simulink model "Imitator_controller"  (R2019b)
settings: Solver=ode4  StartTime=0.0  StopTime=0.6  FixedStep=1e-6  MaxStep=1  RelTol=1e-3  EnableMultiTasking=on
InitFcn:
  | %initialization file
  | clear
  | Rl=0.1;
  | Rload=60;
  | L=2.4e-3;
  | C=14e-6;
  | wref=2*pi*50;
  | Vdc=700;
  | Ts=20e-6;
  | s=tf('s');
  | Vac=325;
  | Td=4e-6;
  | 
  | %net = importKerasNetwork('model_9796.h5','Classes',{'State 1', 'State 2', 'State 3', 'State 4', 'State 5', 'State 6', 'State 7'});
  | %weights1 = double(net.Layers(2,1).Weights);
  | %biases1 = double(net.Layers(2,1).Bias);
  | %weights2 =double(net.Layers(4,1).Weights);
  | %biases2 = double(net.Layers(4,1).Bias);
  | 
  | weights1 = load('weights1.mat');
  | weights1 = weights1.weights1;
  | weights2 = load('weights2.mat');
  | weights2 = weights2.weights2;
  | biases1 = load('biases1.mat');
  | biases1 = biases1.biases1;
  | biases2 = load('biases2.mat');
  | biases2 = biases2.biases2;
undefined symbols (not defined in the file): Lc, Lload, plecs
libraries: neural x95, powerlib x18, powerlib_meascontrol x4
(part 4 of 4)

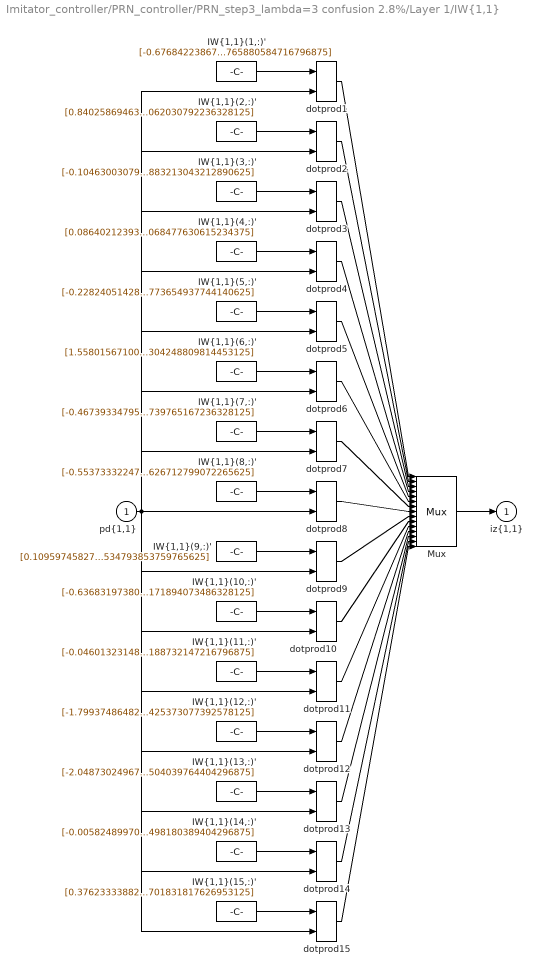
== system Imitator_controller/PRN_controller/PRN_step3_lambda=3 confusion 2.8%/Layer 1/IW{1,1} ==
  "pd{1,1}" : Inport  PortDimensions=8
      mask Display: e = 0.06;c1 = [120 230 180]/255;c2 = ([120 230 180]+0)/(256+128);c3 = ([120 230 180]+128)/(256+128);patch([0 1 1 0],[0 0 1 1],c1);patch([0 1 1 1-e 1-e 0+e],[0 0 1 1-e 0+e 0+e],c2);patch([0 0 1 1-e 0+e 0+e],[0 1 1 1-e 1-e 0+e],c3);plot([0 1 1 0 0],[0 0 1 1 0]);
  "IW{1,1}(1,:)'" : Constant  Value=[-0.676842238677143104297329045948572456836700439453125;-1.9888159175228456998496540109044872224330902099609375;0.73765036780827186735365330605418421328067779541015625;1.71320701226988081344870806788094341754913330078125;0.038398725205589963327401648029990610666573047637939453125;0.04866552570600853055982071282414835877716541290283203125;0.26518608289125467081248643808066844940185546875;-0.19441986416535694814911039429716765880584716796875]
      mask Display: e = 0.06;c1 = [120 150 230]/255;c2 = ([120 150 230]+0)/383;c3 = ([120 150 230]+128)/383;patch([0 1 1 0],[0 0 1 1],c1);patch([0 1 1 1-e 1-e 0+e],[0 0 1 1-e 0+e 0+e],c2);patch([0 0 1 1-e 0+e 0+e],[0 1 1 1-e 1-e 0+e],c3);plot([0 1 1 0 0],[0 0 1 1 0]);disp('Weights');
  "IW{1,1}(10,:)'" : Constant  Value=[-0.63683197380668221665445116741466335952281951904296875;-0.11544459149383486107343088633570005185902118682861328125;-0.36758148612573238178669043918489478528499603271484375;-0.0678774326477270262270025114048621617257595062255859375;-0.046861816789189041088103948595744441263377666473388671875;-0.0058226912142529119176259655432659201323986053466796875;-0.02697450161674534718780904540835763327777385711669921875;1.247120666092144336545288751949556171894073486328125]
      mask Display: e = 0.06;c1 = [120 150 230]/255;c2 = ([120 150 230]+0)/383;c3 = ([120 150 230]+128)/383;patch([0 1 1 0],[0 0 1 1],c1);patch([0 1 1 1-e 1-e 0+e],[0 0 1 1-e 0+e 0+e],c2);patch([0 0 1 1-e 0+e 0+e],[0 1 1 1-e 1-e 0+e],c3);plot([0 1 1 0 0],[0 0 1 1 0]);disp('Weights');
  "IW{1,1}(11,:)'" : Constant  Value=[-0.0460132314806563080811230292965774424374103546142578125;0.01473816958439077250131443719283197424374520778656005859375;0.055555128220495651747423693223026930354535579681396484375;0.049792053782768734560004730838045361451804637908935546875;0.004235491339451513854996722585610768874175846576690673828125;0.003769159624020011235823179873705157660879194736480712890625;-2.82485738553735021838519969605840742588043212890625;-0.01265950989853382828431715978467764216475188732147216796875]
      mask Display: e = 0.06;c1 = [120 150 230]/255;c2 = ([120 150 230]+0)/383;c3 = ([120 150 230]+128)/383;patch([0 1 1 0],[0 0 1 1],c1);patch([0 1 1 1-e 1-e 0+e],[0 0 1 1-e 0+e 0+e],c2);patch([0 0 1 1-e 0+e 0+e],[0 1 1 1-e 1-e 0+e],c3);plot([0 1 1 0 0],[0 0 1 1 0]);disp('Weights');
  "IW{1,1}(12,:)'" : Constant  Value=[-1.7993748648200000861407943375525064766407012939453125;0.1476111476191077909181359473222983069717884063720703125;2.35416836327518108618050973745994269847869873046875;-0.00120452360425208466164492815408948445110581815242767333984375;0.11793391068665191878661602231659344397485256195068359375;0.00113378894210611311406389223321866666083224117755889892578125;1.7721939806664346317433000876917503774166107177734375;-0.268337504582858266122258328323368914425373077392578125]
      mask Display: e = 0.06;c1 = [120 150 230]/255;c2 = ([120 150 230]+0)/383;c3 = ([120 150 230]+128)/383;patch([0 1 1 0],[0 0 1 1],c1);patch([0 1 1 1-e 1-e 0+e],[0 0 1 1-e 0+e 0+e],c2);patch([0 0 1 1-e 0+e 0+e],[0 1 1 1-e 1-e 0+e],c3);plot([0 1 1 0 0],[0 0 1 1 0]);disp('Weights');
  "IW{1,1}(13,:)'" : Constant  Value=[-2.04873024967913952565368163050152361392974853515625;0.1439969197044075333025148211163468658924102783203125;2.577017004086017859521007267176173627376556396484375;0.0318978273732246353500130453539895825088024139404296875;0.11836244796372562271269401890094741247594356536865234375;0.002369781613885219191673048300117443432100117206573486328125;1.8033596226591666056293661313247866928577423095703125;-0.55506848791334906234595791829633526504039764404296875]
      mask Display: e = 0.06;c1 = [120 150 230]/255;c2 = ([120 150 230]+0)/383;c3 = ([120 150 230]+128)/383;patch([0 1 1 0],[0 0 1 1],c1);patch([0 1 1 1-e 1-e 0+e],[0 0 1 1-e 0+e 0+e],c2);patch([0 0 1 1-e 0+e 0+e],[0 1 1 1-e 1-e 0+e],c3);plot([0 1 1 0 0],[0 0 1 1 0]);disp('Weights');
  "IW{1,1}(14,:)'" : Constant  Value=[-0.005824899707417730866654270727167386212386190891265869140625;-0.00300316480099391096281191693151413346640765666961669921875;0.03114520666426491557476907701129675842821598052978515625;0.006670702704397522657397967549286477151326835155487060546875;-0.000317029194644610572660636815811585620394907891750335693359375;-0.0004181329362500792417960127078657706078956834971904754638671875;-4.56994739529403926070472152787260711193084716796875;0.0021206975737620421644524792981201244401745498180389404296875]
      mask Display: e = 0.06;c1 = [120 150 230]/255;c2 = ([120 150 230]+0)/383;c3 = ([120 150 230]+128)/383;patch([0 1 1 0],[0 0 1 1],c1);patch([0 1 1 1-e 1-e 0+e],[0 0 1 1-e 0+e 0+e],c2);patch([0 0 1 1-e 0+e 0+e],[0 1 1 1-e 1-e 0+e],c3);plot([0 1 1 0 0],[0 0 1 1 0]);disp('Weights');
  "IW{1,1}(15,:)'" : Constant  Value=[0.3762333388259329058911362153594382107257843017578125;1.9877672677136974943579161845264025032520294189453125;-0.4572160922242147762517561204731464385986328125;-1.909758831917812482714680299977771937847137451171875;-0.01745565839131461849387250140352989546954631805419921875;-0.07136074826339115773077281801306526176631450653076171875;-1.0942687606048513426770796286291442811489105224609375;0.0170705351700497949540835662673998740501701831817626953125]
      mask Display: e = 0.06;c1 = [120 150 230]/255;c2 = ([120 150 230]+0)/383;c3 = ([120 150 230]+128)/383;patch([0 1 1 0],[0 0 1 1],c1);patch([0 1 1 1-e 1-e 0+e],[0 0 1 1-e 0+e 0+e],c2);patch([0 0 1 1-e 0+e 0+e],[0 1 1 1-e 1-e 0+e],c3);plot([0 1 1 0 0],[0 0 1 1 0]);disp('Weights');
  "IW{1,1}(2,:)'" : Constant  Value=[0.8402586946382888388740184382186271250247955322265625;2.9740480510521773993559691007249057292938232421875;-0.87581495641554429898434364076820202171802520751953125;-2.58606131308167608295889294822700321674346923828125;-0.044568205229961764535229207240263349376618862152099609375;-0.07947286454351652762451152511857799254357814788818359375;-0.41843159002174556970743424244574271142482757568359375;-0.1264744821092489701630512399788131006062030792236328125]
      mask Display: e = 0.06;c1 = [120 150 230]/255;c2 = ([120 150 230]+0)/383;c3 = ([120 150 230]+128)/383;patch([0 1 1 0],[0 0 1 1],c1);patch([0 1 1 1-e 1-e 0+e],[0 0 1 1-e 0+e 0+e],c2);patch([0 0 1 1-e 0+e 0+e],[0 1 1 1-e 1-e 0+e],c3);plot([0 1 1 0 0],[0 0 1 1 0]);disp('Weights');
  "IW{1,1}(3,:)'" : Constant  Value=[-0.10463003079453410404386914933638763613998889923095703125;-0.148811432180895708565770974018960259854793548583984375;0.3554158485937028988388419747934676706790924072265625;0.733725620377389642357002230710349977016448974609375;0.01469423798528121140327673543879427597858011722564697265625;0.04790304967176783890181468450464308261871337890625;0.2803715055990263493868042132817208766937255859375;-0.59524025998255414293680587434209883213043212890625]
      mask Display: e = 0.06;c1 = [120 150 230]/255;c2 = ([120 150 230]+0)/383;c3 = ([120 150 230]+128)/383;patch([0 1 1 0],[0 0 1 1],c1);patch([0 1 1 1-e 1-e 0+e],[0 0 1 1-e 0+e 0+e],c2);patch([0 0 1 1-e 0+e 0+e],[0 1 1 1-e 1-e 0+e],c3);plot([0 1 1 0 0],[0 0 1 1 0]);disp('Weights');
  "IW{1,1}(4,:)'" : Constant  Value=[0.08640212393146283476053071126443683169782161712646484375;-0.332422172544865890397858265714603476226329803466796875;0.134396737678882105537780944359838031232357025146484375;-0.466363177669556983051535326012526638805866241455078125;0.009933573064589286405468016027953126467764377593994140625;-0.03107822960809668300097285964511684142053127288818359375;0.11826162876171357474230916295709903351962566375732421875;-0.6759966479300183461731421630247496068477630615234375]
      mask Display: e = 0.06;c1 = [120 150 230]/255;c2 = ([120 150 230]+0)/383;c3 = ([120 150 230]+128)/383;patch([0 1 1 0],[0 0 1 1],c1);patch([0 1 1 1-e 1-e 0+e],[0 0 1 1-e 0+e 0+e],c2);patch([0 0 1 1-e 0+e 0+e],[0 1 1 1-e 1-e 0+e],c3);plot([0 1 1 0 0],[0 0 1 1 0]);disp('Weights');
  "IW{1,1}(5,:)'" : Constant  Value=[-0.228240514285129869609392017082427628338336944580078125;-0.11942127931433177412401391848106868565082550048828125;-0.5189150642454960493665794274420477449893951416015625;-0.2180770107122695922186039751977659761905670166015625;-0.0435788874720391683492692891377373598515987396240234375;-0.01491340110063483527513827908705934532918035984039306640625;-0.15095191620441905655525260954163968563079833984375;-0.782450803183126541995306979515589773654937744140625]
      mask Display: e = 0.06;c1 = [120 150 230]/255;c2 = ([120 150 230]+0)/383;c3 = ([120 150 230]+128)/383;patch([0 1 1 0],[0 0 1 1],c1);patch([0 1 1 1-e 1-e 0+e],[0 0 1 1-e 0+e 0+e],c2);patch([0 0 1 1-e 0+e 0+e],[0 1 1 1-e 1-e 0+e],c3);plot([0 1 1 0 0],[0 0 1 1 0]);disp('Weights');
  "IW{1,1}(6,:)'" : Constant  Value=[1.558015671008904146077611585496924817562103271484375;-0.1180797300911171909820751579900388605892658233642578125;-1.902660599685177533757496348698623478412628173828125;0.003977377146006866141803026692969069699756801128387451171875;-0.08348369673845212890483935552765615284442901611328125;0.0026863952881113427849368857636136453947983682155609130859375;-1.4000784832777390942482043101335875689983367919921875;0.39625979900872654315691079318639822304248809814453125]
      mask Display: e = 0.06;c1 = [120 150 230]/255;c2 = ([120 150 230]+0)/383;c3 = ([120 150 230]+128)/383;patch([0 1 1 0],[0 0 1 1],c1);patch([0 1 1 1-e 1-e 0+e],[0 0 1 1-e 0+e 0+e],c2);patch([0 0 1 1-e 0+e 0+e],[0 1 1 1-e 1-e 0+e],c3);plot([0 1 1 0 0],[0 0 1 1 0]);disp('Weights');
  "IW{1,1}(7,:)'" : Constant  Value=[-0.46739334795190135007914022935437969863414764404296875;2.178515494617806691479700020863674581050872802734375;0.6448005482874654692437843550578691065311431884765625;-1.9184457260679244061662984677241183817386627197265625;0.0294271182263212312257838476625693147070705890655517578125;-0.0623981982945895630177091106816078536212444305419921875;0.61248428221931672243982802683603949844837188720703125;0.067143770619634779439621752317179925739765167236328125]
      mask Display: e = 0.06;c1 = [120 150 230]/255;c2 = ([120 150 230]+0)/383;c3 = ([120 150 230]+128)/383;patch([0 1 1 0],[0 0 1 1],c1);patch([0 1 1 1-e 1-e 0+e],[0 0 1 1-e 0+e 0+e],c2);patch([0 0 1 1-e 0+e 0+e],[0 1 1 1-e 1-e 0+e],c3);plot([0 1 1 0 0],[0 0 1 1 0]);disp('Weights');
  "IW{1,1}(8,:)'" : Constant  Value=[-0.5537333224702154499397011022665537893772125244140625;2.2076507516497034799840548657812178134918212890625;0.71130173728132450872152503507095389068126678466796875;-1.8325370125449389480110085060005076229572296142578125;0.032513497429587888409852070026317960582673549652099609375;-0.0567763705086160863633182316334568895399570465087890625;0.7079486893093649424457680652267299592494964599609375;-0.195914278192344915030531637967214919626712799072265625]
      mask Display: e = 0.06;c1 = [120 150 230]/255;c2 = ([120 150 230]+0)/383;c3 = ([120 150 230]+128)/383;patch([0 1 1 0],[0 0 1 1],c1);patch([0 1 1 1-e 1-e 0+e],[0 0 1 1-e 0+e 0+e],c2);patch([0 0 1 1-e 0+e 0+e],[0 1 1 1-e 1-e 0+e],c3);plot([0 1 1 0 0],[0 0 1 1 0]);disp('Weights');
  "IW{1,1}(9,:)'" : Constant  Value=[0.10959745827120991046310649608130916021764278411865234375;-0.1151261666569428354645054923821589909493923187255859375;0.238238515218123503291991482910816557705402374267578125;-0.599483509913133705282461960450746119022369384765625;0.0182118939746620071840066401591684552840888500213623046875;-0.040196607461508417069584453429342829622328281402587890625;0.257225616068732787500294989513349719345569610595703125;0.74979559802271344981505762916640378534793853759765625]
      mask Display: e = 0.06;c1 = [120 150 230]/255;c2 = ([120 150 230]+0)/383;c3 = ([120 150 230]+128)/383;patch([0 1 1 0],[0 0 1 1],c1);patch([0 1 1 1-e 1-e 0+e],[0 0 1 1-e 0+e 0+e],c2);patch([0 0 1 1-e 0+e 0+e],[0 1 1 1-e 1-e 0+e],c3);plot([0 1 1 0 0],[0 0 1 1 0]);disp('Weights');
  Mux : Mux  Inputs=15
      mask Display: e = 0.06;c1 = [120 150 230]/255;c2 = ([120 150 230]+0)/383;c3 = ([120 150 230]+128)/383;patch([0 1 1 0],[0 0 1 1],c1);patch([0 1 1 1-e 1-e 0+e],[0 0 1 1-e 0+e 0+e],c2);patch([0 0 1 1-e 0+e 0+e],[0 1 1 1-e 1-e 0+e],c3);plot([0 1 1 0 0],[0 0 1 1 0]);disp('Mux');
  dotprod{1..15} (15 alike) : neural/Weight Functions/dotprod
      settings: SourceProductName=Deep Learning Toolbox
  "iz{1,1}" : Outport  VectorParamsAs1DForOutWhenUnconnected=off
      mask Display: e = 0.06;c1 = [120 230 180]/255;c2 = ([120 230 180]+0)/(256+128);c3 = ([120 230 180]+128)/(256+128);patch([0 1 1 0],[0 0 1 1],c1);patch([0 1 1 1-e 1-e 0+e],[0 0 1 1-e 0+e 0+e],c2);patch([0 0 1 1-e 0+e 0+e],[0 1 1 1-e 1-e 0+e],c3);plot([0 1 1 0 0],[0 0 1 1 0]);
  wires:
  "IW{1,1}(1,:)'"/1 -> dotprod1/1
  "pd{1,1}"/1 -> dotprod1/2, dotprod2/2, dotprod3/2, dotprod4/2, dotprod5/2, dotprod6/2, dotprod7/2, dotprod8/2, dotprod9/2, dotprod10/2, dotprod11/2, dotprod12/2, dotprod13/2, dotprod14/2, dotprod15/2
  dotprod1/1 -> Mux/1
  "IW{1,1}(2,:)'"/1 -> dotprod2/1
  dotprod2/1 -> Mux/2
  "IW{1,1}(3,:)'"/1 -> dotprod3/1
  dotprod3/1 -> Mux/3
  "IW{1,1}(4,:)'"/1 -> dotprod4/1
  dotprod4/1 -> Mux/4
  "IW{1,1}(5,:)'"/1 -> dotprod5/1
  dotprod5/1 -> Mux/5
  "IW{1,1}(6,:)'"/1 -> dotprod6/1
  dotprod6/1 -> Mux/6
  "IW{1,1}(7,:)'"/1 -> dotprod7/1
  dotprod7/1 -> Mux/7
  "IW{1,1}(8,:)'"/1 -> dotprod8/1
  dotprod8/1 -> Mux/8
  "IW{1,1}(9,:)'"/1 -> dotprod9/1
  dotprod9/1 -> Mux/9
  "IW{1,1}(10,:)'"/1 -> dotprod10/1
  dotprod10/1 -> Mux/10
  "IW{1,1}(11,:)'"/1 -> dotprod11/1
  dotprod11/1 -> Mux/11
  "IW{1,1}(12,:)'"/1 -> dotprod12/1
  dotprod12/1 -> Mux/12
  "IW{1,1}(13,:)'"/1 -> dotprod13/1
  dotprod13/1 -> Mux/13
  "IW{1,1}(14,:)'"/1 -> dotprod14/1
  dotprod14/1 -> Mux/14
  "IW{1,1}(15,:)'"/1 -> dotprod15/1
  dotprod15/1 -> Mux/15
  Mux/1 -> "iz{1,1}"/1

== system Imitator_controller/PRN_controller/PRN_step3_lambda=3 confusion 2.8%/Layer 2/Delays 1 ==
  "p{2}" : Inport  PortDimensions=15
      mask Display: e = 0.06;c1 = [120 230 180]/255;c2 = ([120 230 180]+0)/(256+128);c3 = ([120 230 180]+128)/(256+128);patch([0 1 1 0],[0 0 1 1],c1);patch([0 1 1 1-e 1-e 0+e],[0 0 1 1-e 0+e 0+e],c2);patch([0 0 1 1-e 0+e 0+e],[0 1 1 1-e 1-e 0+e],c3);plot([0 1 1 0 0],[0 0 1 1 0]);
  mux : Mux  Inputs=1
      mask Display: e = 0.06;c1 = [120 150 230]/255;c2 = ([120 150 230]+0)/383;c3 = ([120 150 230]+128)/383;patch([0 1 1 0],[0 0 1 1],c1);patch([0 1 1 1-e 1-e 0+e],[0 0 1 1-e 0+e 0+e],c2);patch([0 0 1 1-e 0+e 0+e],[0 1 1 1-e 1-e 0+e],c3);plot([0 1 1 0 0],[0 0 1 1 0]);disp('Mux')
  "pd{2,1}" : Outport  VectorParamsAs1DForOutWhenUnconnected=off
      mask Display: e = 0.06;c1 = [120 230 180]/255;c2 = ([120 230 180]+0)/(256+128);c3 = ([120 230 180]+128)/(256+128);patch([0 1 1 0],[0 0 1 1],c1);patch([0 1 1 1-e 1-e 0+e],[0 0 1 1-e 0+e 0+e],c2);patch([0 0 1 1-e 0+e 0+e],[0 1 1 1-e 1-e 0+e],c3);plot([0 1 1 0 0],[0 0 1 1 0]);
  wires:
  "p{2}"/1 -> mux/1
  mux/1 -> "pd{2,1}"/1

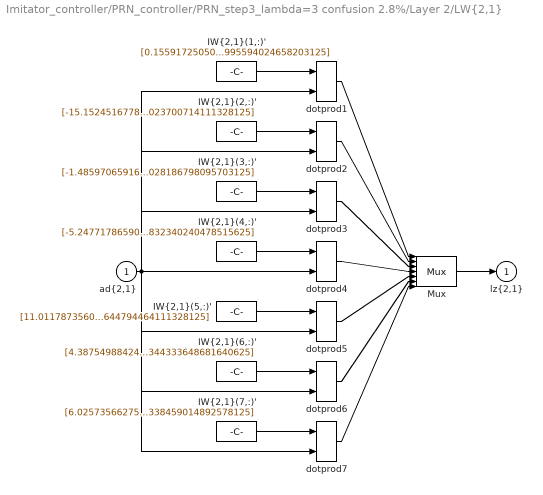
== system Imitator_controller/PRN_controller/PRN_step3_lambda=3 confusion 2.8%/Layer 2/LW{2,1} ==
  "ad{2,1}" : Inport  PortDimensions=15
      mask Display: e = 0.06;c1 = [120 230 180]/255;c2 = ([120 230 180]+0)/(256+128);c3 = ([120 230 180]+128)/(256+128);patch([0 1 1 0],[0 0 1 1],c1);patch([0 1 1 1-e 1-e 0+e],[0 0 1 1-e 0+e 0+e],c2);patch([0 0 1 1-e 0+e 0+e],[0 1 1 1-e 1-e 0+e],c3);plot([0 1 1 0 0],[0 0 1 1 0]);
  "IW{2,1}(1,:)'" : Constant  Value=[0.1559172505041254430668828945272252894937992095947265625;-1.0015595831774444235406917869113385677337646484375;0.66080340506745860462700647985911928117275238037109375;-0.6120871928899653813260783863370306789875030517578125;0.205693335569471280610542862632428295910358428955078125;0.460691248027044253365858139659394510090351104736328125;0.16527146808664860966331389136030338704586029052734375;-0.437118286681691781137004682022961787879467010498046875;0.038940007239061158461623790572048164904117584228515625;0.2361328917164233487380187170856515876948833465576171875;-0.382518092552544874962450194288976490497589111328125;-0.00145317437137639469957317572834654129110276699066162109375;-0.01496688930234552593334651504619614570401608943939208984375;-0.045107306904926321167170755188635666854679584503173828125;0.393169879516289899612502267700619995594024658203125]
      mask Display: e = 0.06;c1 = [120 150 230]/255;c2 = ([120 150 230]+0)/383;c3 = ([120 150 230]+128)/383;patch([0 1 1 0],[0 0 1 1],c1);patch([0 1 1 1-e 1-e 0+e],[0 0 1 1-e 0+e 0+e],c2);patch([0 0 1 1-e 0+e 0+e],[0 1 1 1-e 1-e 0+e],c3);plot([0 1 1 0 0],[0 0 1 1 0]);disp('weights');
  "IW{2,1}(2,:)'" : Constant  Value=[-15.1524516778410234252305599511601030826568603515625;7.62661201024433399453528181766159832477569580078125;-7.08578304485774967957922854111529886722564697265625;-6.307827169387355326080069062300026416778564453125;13.276742462632324048854570719413459300994873046875;8.4202039847483973744601826183497905731201171875;-13.158769761155927113804864347912371158599853515625;-15.5715647022098817586766017484478652477264404296875;-6.72812882018975866316168321645818650722503662109375;-9.03835274223421691885960171930491924285888671875;-19.01903941784602380948854261077940464019775390625;-10.4829189851118673715291151893325150012969970703125;-8.4056388180317611613645567558705806732177734375;-16.08709361177763952355235232971608638763427734375;4.6153368959157194950648772646673023700714111328125]
      mask Display: e = 0.06;c1 = [120 150 230]/255;c2 = ([120 150 230]+0)/383;c3 = ([120 150 230]+128)/383;patch([0 1 1 0],[0 0 1 1],c1);patch([0 1 1 1-e 1-e 0+e],[0 0 1 1-e 0+e 0+e],c2);patch([0 0 1 1-e 0+e 0+e],[0 1 1 1-e 1-e 0+e],c3);plot([0 1 1 0 0],[0 0 1 1 0]);disp('weights');
  "IW{2,1}(3,:)'" : Constant  Value=[-1.485970659162996643232190763228572905063629150390625;4.40404883137724656450018301256932318210601806640625;-8.524713265715593735194488544948399066925048828125;9.5853062598504710223323854734189808368682861328125;12.68294592043289270577588467858731746673583984375;10.848054732692073542921207263134419918060302734375;10.134655139995413009046387742273509502410888671875;7.4394578313788546353180208825506269931793212890625;7.00835588390813502002174573135562241077423095703125;-6.4881605392343804084021030575968325138092041015625;-24.051609846023151106919613084755837917327880859375;-10.643350217411178704196572653017938137054443359375;-10.4188066070471077040338059305213391780853271484375;1.812415352920940136982608237303793430328369140625;6.7111848631215327287691252422519028186798095703125]
      mask Display: e = 0.06;c1 = [120 150 230]/255;c2 = ([120 150 230]+0)/383;c3 = ([120 150 230]+128)/383;patch([0 1 1 0],[0 0 1 1],c1);patch([0 1 1 1-e 1-e 0+e],[0 0 1 1-e 0+e 0+e],c2);patch([0 0 1 1-e 0+e 0+e],[0 1 1 1-e 1-e 0+e],c3);plot([0 1 1 0 0],[0 0 1 1 0]);disp('weights');
  "IW{2,1}(4,:)'" : Constant  Value=[-5.247717865902817635515020810998976230621337890625;5.42662020212826678999817886506207287311553955078125;-5.20147797786081245163813946419395506381988525390625;15.8895682575992598373204600648023188114166259765625;-4.0853051369030755068934013252146542072296142578125;-10.18706059702028454694300307892262935638427734375;7.93839020767507275166963154333643615245819091796875;7.37595380569916159174681524746119976043701171875;12.7459665360532437006213513086549937725067138671875;5.39319027560176156299576177843846380710601806640625;-3.993536637098486163921506886254064738750457763671875;10.8577061634513842847127307322807610034942626953125;9.992983141235800559343260829336941242218017578125;20.42069020795066336404488538391888141632080078125;3.921999546686420590191346491337753832340240478515625]
      mask Display: e = 0.06;c1 = [120 150 230]/255;c2 = ([120 150 230]+0)/383;c3 = ([120 150 230]+128)/383;patch([0 1 1 0],[0 0 1 1],c1);patch([0 1 1 1-e 1-e 0+e],[0 0 1 1-e 0+e 0+e],c2);patch([0 0 1 1-e 0+e 0+e],[0 1 1 1-e 1-e 0+e],c3);plot([0 1 1 0 0],[0 0 1 1 0]);disp('weights');
  "IW{2,1}(5,:)'" : Constant  Value=[11.01178735609996550692812888883054256439208984375;-9.9278819178309891668732234393246471881866455078125;8.401288431422376135060403612442314624786376953125;5.1970715821688298063918409752659499645233154296875;-12.4478749824383694289053892134688794612884521484375;-9.280564902142717897959300898946821689605712890625;13.42498613067466095571944606490433216094970703125;10.1908309194200672465058232774026691913604736328125;7.9773842034973636572203758987598121166229248046875;9.3408347915467491162644364521838724613189697265625;17.651254466441724133574098232202231884002685546875;11.4345043923240670125096585252322256565093994140625;10.4974967832880725637778596137650310993194580078125;15.47662651006276490761592867784202098846435546875;-1.28812184262068729623251783777959644794464111328125]
      mask Display: e = 0.06;c1 = [120 150 230]/255;c2 = ([120 150 230]+0)/383;c3 = ([120 150 230]+128)/383;patch([0 1 1 0],[0 0 1 1],c1);patch([0 1 1 1-e 1-e 0+e],[0 0 1 1-e 0+e 0+e],c2);patch([0 0 1 1-e 0+e 0+e],[0 1 1 1-e 1-e 0+e],c3);plot([0 1 1 0 0],[0 0 1 1 0]);disp('weights');
  "IW{2,1}(6,:)'" : Constant  Value=[4.38754988424871417151962305069901049137115478515625;-4.51435816810777179597380381892435252666473388671875;9.42502334521616802476273733191192150115966796875;-9.85131454862557376372933504171669483184814453125;-11.5816907193186384716909742564894258975982666015625;-9.2017607375453689400046641821973025798797607421875;-8.8048528080077854696128270006738603115081787109375;-6.21533510273211842189766684896312654018402099609375;-6.3681023049225959908881122828461229801177978515625;5.61746976164818878629603204899467527866363525390625;23.847661371737554958372129476629197597503662109375;9.8113737143322286016200450831092894077301025390625;9.749795149296847540654198382981121540069580078125;-1.1155165722736370970125108215142972767353057861328125;-7.73127435709400234742361135431565344333648681640625]
      mask Display: e = 0.06;c1 = [120 150 230]/255;c2 = ([120 150 230]+0)/383;c3 = ([120 150 230]+128)/383;patch([0 1 1 0],[0 0 1 1],c1);patch([0 1 1 1-e 1-e 0+e],[0 0 1 1-e 0+e 0+e],c2);patch([0 0 1 1-e 0+e 0+e],[0 1 1 1-e 1-e 0+e],c3);plot([0 1 1 0 0],[0 0 1 1 0]);disp('weights');
  "IW{2,1}(7,:)'" : Constant  Value=[6.02573566275810179604377481155097484588623046875;-5.6208227016348946136758968350477516651153564453125;3.4599191770390387290490252780728042125701904296875;-15.0713212579686217651442348142154514789581298828125;2.728270614810654581816606878419406712055206298828125;10.9215647698604758630835931398905813694000244140625;-8.4335005707785040129920162144117057323455810546875;-4.90550296610703373545447902870364487171173095703125;-14.838916323974640221194931655190885066986083984375;-5.95385456154587533461608472862280905246734619140625;4.3334765344362775607578441849909722805023193359375;-11.285309454955854135960180428810417652130126953125;-10.8122696962447495394599172868765890598297119140625;-19.91277132590794707311943056993186473846435546875;-6.9656592292055439230580304865725338459014892578125]
      mask Display: e = 0.06;c1 = [120 150 230]/255;c2 = ([120 150 230]+0)/383;c3 = ([120 150 230]+128)/383;patch([0 1 1 0],[0 0 1 1],c1);patch([0 1 1 1-e 1-e 0+e],[0 0 1 1-e 0+e 0+e],c2);patch([0 0 1 1-e 0+e 0+e],[0 1 1 1-e 1-e 0+e],c3);plot([0 1 1 0 0],[0 0 1 1 0]);disp('weights');
  Mux : Mux  Inputs=7
      mask Display: e = 0.06;c1 = [120 150 230]/255;c2 = ([120 150 230]+0)/383;c3 = ([120 150 230]+128)/383;patch([0 1 1 0],[0 0 1 1],c1);patch([0 1 1 1-e 1-e 0+e],[0 0 1 1-e 0+e 0+e],c2);patch([0 0 1 1-e 0+e 0+e],[0 1 1 1-e 1-e 0+e],c3);plot([0 1 1 0 0],[0 0 1 1 0]);disp('Mux');
  dotprod{1..7} (7 alike) : neural/Weight Functions/dotprod
      settings: SourceProductName=Deep Learning Toolbox
  "lz{2,1}" : Outport  VectorParamsAs1DForOutWhenUnconnected=off
      mask Display: e = 0.06;c1 = [120 230 180]/255;c2 = ([120 230 180]+0)/(256+128);c3 = ([120 230 180]+128)/(256+128);patch([0 1 1 0],[0 0 1 1],c1);patch([0 1 1 1-e 1-e 0+e],[0 0 1 1-e 0+e 0+e],c2);patch([0 0 1 1-e 0+e 0+e],[0 1 1 1-e 1-e 0+e],c3);plot([0 1 1 0 0],[0 0 1 1 0]);
  wires:
  "IW{2,1}(1,:)'"/1 -> dotprod1/1
  "ad{2,1}"/1 -> dotprod1/2, dotprod2/2, dotprod3/2, dotprod4/2, dotprod5/2, dotprod6/2, dotprod7/2
  dotprod1/1 -> Mux/1
  "IW{2,1}(2,:)'"/1 -> dotprod2/1
  dotprod2/1 -> Mux/2
  "IW{2,1}(3,:)'"/1 -> dotprod3/1
  dotprod3/1 -> Mux/3
  "IW{2,1}(4,:)'"/1 -> dotprod4/1
  dotprod4/1 -> Mux/4
  "IW{2,1}(5,:)'"/1 -> dotprod5/1
  dotprod5/1 -> Mux/5
  "IW{2,1}(6,:)'"/1 -> dotprod6/1
  dotprod6/1 -> Mux/6
  "IW{2,1}(7,:)'"/1 -> dotprod7/1
  dotprod7/1 -> Mux/7
  Mux/1 -> "lz{2,1}"/1

== matlab function Imitator_controller/PRN_controller/  ==
  settings: sampleTime=33*1e-6
  data: SW_out output double size=[1 3] [0..1]; class input double; x_old output
function [SW_out, x_old]=output(class)

vector= [0 0 0; 1 0 0; 1 1 0; 0 1 0; 0 1 1; 0 0 1; 1 0 1];

x_old = 1; % initialization

sw_min = zeros(1,3);
if class(1) == 1
    sw_min = vector(1,:);
    x_old = 1;
elseif class(2) == 1
    sw_min = vector(2,:);
    x_old = 2;
elseif class(3) == 1
    sw_min = vector(3,:);
    x_old = 3;
elseif class(4) == 1
    sw_min = vector(4,:);
    x_old = 4;
elseif class(5) == 1
    sw_min = vector(5,:);
    x_old = 5;
elseif class(6) == 1
    sw_min = vector(6,:);
     x_old = 6;
elseif class(7) == 1
    sw_min = vector(7,:);
    x_old = 7;
elseif isempty(class)    
    sw_min = vector(randi([1 7],1,1),:);
    x_old = 1;
end

SW_out=[sw_min];

== matlab function Imitator_controller/Avg. freq calculation/MATLAB Function ==
  data: S_old input; sw output; S_new input
function sw = fcn(S_old, S_new)

sw = sum(abs(S_old(1,:)-S_new(1,:)));

== matlab function Imitator_controller/PRN_controller/Input data vector generation ==
  settings: sampleTime=33*1e-6
  data: InputPaper output; v_meas_alpha input; v_meas_beta input; i_meas_alpha input; i_meas_beta input; v_ref_alpha input; v_ref_beta input; i_load_alpha input; i_load_beta input; x_old input; Input output
function [InputPaper, Input] = measurements(v_meas_alpha,v_meas_beta, i_meas_alpha,i_meas_beta, v_ref_alpha, v_ref_beta, i_load_alpha, i_load_beta, x_old)

delta_Vc_alpha = v_meas_alpha - v_ref_alpha;  
delta_Vc_beta =  v_meas_beta - v_ref_beta;

R1 = sqrt(v_meas_alpha^2 +  v_meas_beta^2)/sqrt(i_load_alpha^2 + i_load_beta^2); 

InputPaper = [v_ref_alpha, v_ref_beta, i_meas_alpha, i_meas_beta, delta_Vc_alpha, delta_Vc_beta, x_old, R1]';
Input = [R1, i_meas_alpha, i_meas_beta, delta_Vc_alpha, delta_Vc_beta, v_ref_alpha, v_ref_beta, x_old]';

== matlab function Imitator_controller/PRN_controller/MATLAB Function1 ==
  data: input_data input; SW_out output; sw_freq output; weights1 input; biases1 input; weights2 input; biases2 input; x_old output
function [SW_out, sw_freq, x_old] = neural_network(input_data, weights1, biases1, weights2, biases2)

layer1 = relu(weights1*input_data + biases1);
layer2 = weights2*layer1 + biases2;
%layer2 = softmax(weights2*layer1 + biases2);

    function y = relu(x)
        y = zeros(length(x),1);
        for i = 1:length(x)
            if x(i) > 0 
                y(i) = x(i);
            else
                y(i) = 0;
            end
        end
    end

%     function y = softmax(x)
%         den = sum(exp(x));
%         y = zeros(length(x),1);
%         for i = 1:length(x)
%             y(i) = exp(x(i))/den;
%         end
%     end

[~,opt_state] = max(layer2);

vector= [0 0 0; 1 0 0; 1 1 0; 0 1 0; 0 1 1; 0 0 1; 1 0 1];

SW_out = vector(opt_state,:)';
sw_freq=SW_out';
x_old = opt_state;

end
